simulink model "testFIB"  (R2021a)
settings: Solver=FixedStepAuto  StartTime=0.0  StopTime=20  RelTol=1e-3
undefined symbols (not defined in the file or in its folder): at, Stuck
libraries: FIBlockLib x2
settings Model: Creator=flata  LastModifiedBy=DELL
settings SolverCC: AlgebraicLoopSolver=TrustRegion
settings DebuggingCC: SFMachineParentedDataDiag=warning

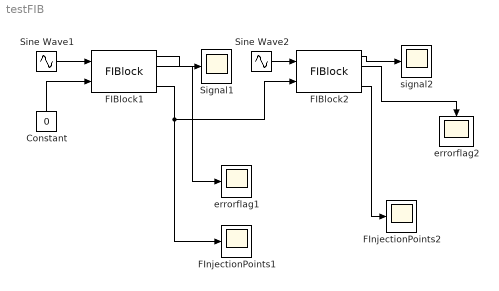
== system testFIB ==
  Constant : Constant  Value=0
  FIBlock1 : FIBlockLib/FIBlock  FIBlockName=1  FInjEnable=on  FaultType=Time delay  FaultValue=40  FaultEvent=Deterministic  EventValue=5  FaultEffect=Constant time  EffectValue=2
      settings: SourceProductName=Fault Injection block
  FIBlock2 : FIBlockLib/FIBlock  FIBlockName=2  FInjEnable=on  FaultType=Stuck-at  FaultValue=2  FaultEvent=Deterministic  EventValue=9  FaultEffect=Once  EffectValue=0
      settings: SourceProductName=Fault Injection block
  FInjectionPoints1 : Scope
  FInjectionPoints2 : Scope
  Signal1 : Scope
  Sine Wave1 : Sin  SampleTime=0
  Sine Wave2 : Sin  SampleTime=0
  errorflag1 : Scope
  errorflag2 : Scope
  signal2 : Scope
  wires:
  FIBlock2/1 -> signal2/1
  FIBlock2/2 -> errorflag2/1
  Sine Wave2/1 -> FIBlock2/1
  FIBlock1/1 -> Signal1/1
  Constant/1 -> FIBlock1/2
  Sine Wave1/1 -> FIBlock1/1
  FIBlock1/2 -> errorflag1/1
  FIBlock1/4 -> FIBlock2/2, FInjectionPoints1/1
  FIBlock2/4 -> FInjectionPoints2/1
